simulink model "simulinktp1"  (R2026a)
settings: Solver=VariableStepAuto  StopTime=2000
settings Model: Creator=21414298  LastModifiedBy=21414298

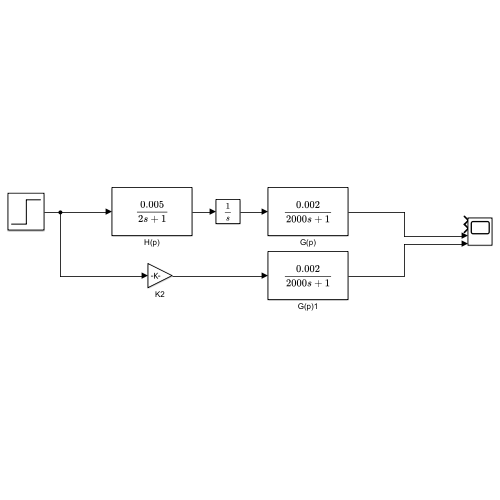
[thumbnail: Simulink's stored preview of the top-level diagram]
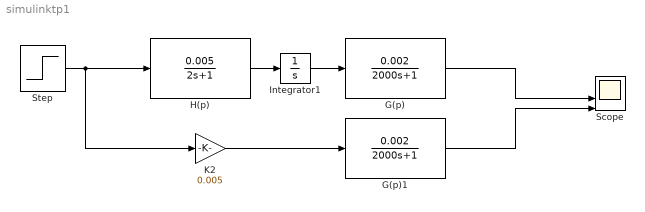
== system simulinktp1 ==
  G(p) : TransferFcn  Numerator=[0.002]  Denominator=[2000 1]
  G(p)1 : TransferFcn  Numerator=[0.002]  Denominator=[2000 1]
  H(p) : TransferFcn  Numerator=[0.005]  Denominator=[2 1]
  Integrator1 : Integrator
  K2 : Gain  Gain=0.005
  Scope : Scope  NumInputPorts=4
      settings: ActiveDisplayYMinimum=-7.8992071639422081E-7  ActiveDisplayYMaximum=7.1092864475479892E-6
  Step : Step  SampleTime=0
  wires:
  Step/1 -> K2/1, H(p)/1
  Integrator1/1 -> G(p)/1
  H(p)/1 -> Integrator1/1
  K2/1 -> G(p)1/1
  G(p)/1 -> Scope/3
  G(p)1/1 -> Scope/4
